simulink model "sm_controlled_current_boost_modificado_renan"  (R2016a)
settings: Solver=VariableStepAuto  StartTime=0.0  StopTime=5  RelTol=1e-3
libraries: powerlib x12
settings Model: Creator=jorda  LastModifiedBy=jorda

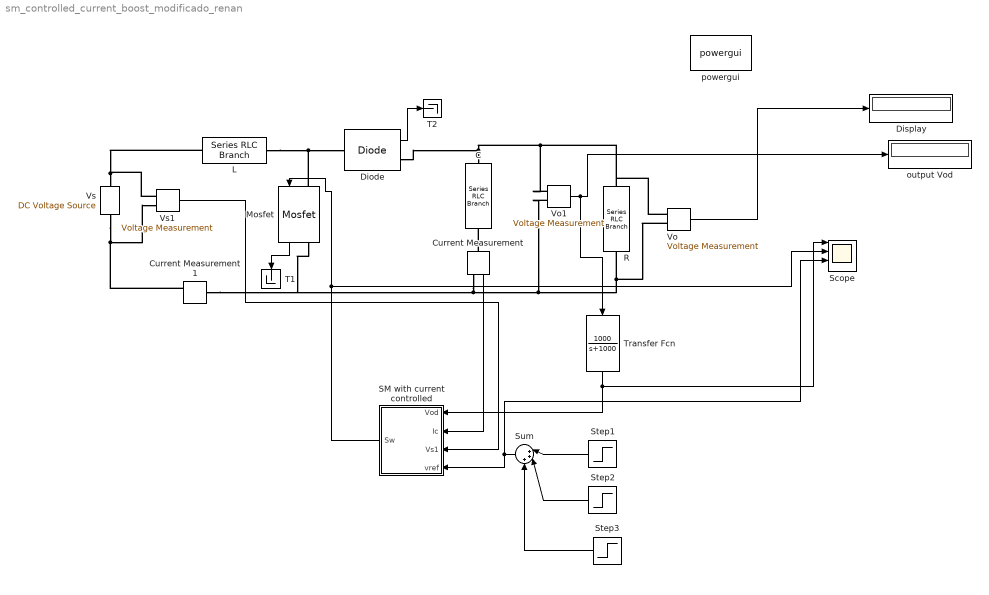
== system sm_controlled_current_boost_modificado_renan ==
  C : powerlib/Elements/Series RLC Branch  LConnTagsString=__new0  RConnTagsString=__new0  BranchType=C  Resistance=1  Inductance=1e-3  SetiL0=off  InitialCurrent=0  Capacitance=2000e-6  Setx0=off  InitialVoltage=0  Measurements=None
  Current Measurement : powerlib/Measurements/Current Measurement  PhasorSimulation=off  OutputType=Complex  PSBequivalent=0
  Current Measurement1 : powerlib/Measurements/Current Measurement  PhasorSimulation=off  OutputType=Complex  PSBequivalent=0
  Diode : powerlib/Power Electronics/Diode  Ron=0.001  Lon=0  Vf=0.8  IC=0  UseSnubber=off  Rs=500  Cs=250e-9  Measurements=on
  Display : Display
  L : powerlib/Elements/Series RLC Branch  LConnTagsString=__new0  RConnTagsString=__new0  BranchType=L  Resistance=1  Inductance=2e-3  SetiL0=off  InitialCurrent=0  Capacitance=1e-6  Setx0=off  InitialVoltage=0  Measurements=None
  Mosfet : powerlib/Power Electronics/Mosfet  Ron=0.1  Lon=0  Rd=0.01  Vfd=0  IC=0  Rs=1e5  Cs=inf  Measurements=on
  R : powerlib/Elements/Series RLC Branch  LConnTagsString=__new0  RConnTagsString=__new0  BranchType=R  Resistance=4  Inductance=1e-3  SetiL0=off  InitialCurrent=0  Capacitance=1e-6  Setx0=off  InitialVoltage=0  Measurements=None
  SM with current controlled : Subsystem
  Scope : Scope  NumInputPorts=4
  Step1 : Step  Before=20  After=22  SampleTime=0
  Step2 : Step  Time=3  After=-2  SampleTime=0
  Step3 : Step  Time=4  Before=3  After=0  SampleTime=0
  Sum : Sum  Inputs=|+++
  T1 : Terminator
  T2 : Terminator
  Transfer Fcn : TransferFcn  Numerator=[1000]  Denominator=[1 1000]
  Vo : powerlib/Measurements/Voltage Measurement  PhasorSimulation=off  OutputType=Complex  PSBequivalent=0
  Vo1 : powerlib/Measurements/Voltage Measurement  PhasorSimulation=off  OutputType=Complex  PSBequivalent=0
  Vs : powerlib/Electrical Sources/DC Voltage Source  Amplitude=15  Measurements=None
  Vs1 : powerlib/Measurements/Voltage Measurement  PhasorSimulation=off  OutputType=Complex  PSBequivalent=0
  output Vod : Display
  powergui : powerlib/powergui  Priority=1  SimulationMode=Continuous  SolverType=Tustin/Backward Euler (TBE)  SampleTime=50e-6  frequency=60  SPID=off  DisableSnubberDevices=off  DisableRonSwitches=off  DisableVfSwitches=off  SwTol=0  DisplayEquations=off  Interpol=off  ExternalGateDelay=off  methode=off  Ts=10  FunctionMessages=off  echomessages=off  HookPort=off  EnableUseOfTLC=off  x0status=blocks  frequencyindice=0  Pbase=100e6  ErrMax=1e-4  Iterations=50  UnitsV=kV  UnitsW=MW  buscounter=0  RestoreLinks=warning  ResistiveCurrentMeasurement=off  Frange=[0:2:500]  Ylog=off  Xlog=on  ShowGrid=off  save=off  variable=ZData  structure=0  ZoomFFT=off  StartTime=0.0  cycles=1  DisplayStyle=1  fundamental=60  FreqAxis=off  MaxFrequency=1000  frequencyindicesteady=1  RmsSteady=1  display=off
  wires:
  Mosfet/1 -> T1/1
  Current Measurement/1 -> SM with current controlled/2(Ic)
  Diode/1 -> T2/1
  SM with current controlled/1(Sw) -> Mosfet/1, Scope/2
  Vs1/1 -> SM with current controlled/3("Vs1 ")
  Step1/1 -> Sum/1
  Sum/1 -> Scope/3, SM with current controlled/4(vref)
  Step2/1 -> Sum/2
  Vo/1 -> Display/1
  Vo1/1 -> Transfer Fcn/1, output Vod/1
  Transfer Fcn/1 -> Scope/1, SM with current controlled/1(Vod)
  Step3/1 -> Sum/3
  connections:
  R/LConn1 -- Vo/LConn1 -- Vo1/LConn1 -- Diode/RConn1 -- C/LConn1
  Current Measurement/RConn1 -- Current Measurement1/LConn1 -- Mosfet/RConn1 -- Vo1/LConn2 -- R/RConn1 -- Vo/LConn2
  Current Measurement/LConn1 -- C/RConn1
  L/RConn1 -- Mosfet/LConn1 -- Diode/LConn1
  Vs/RConn1 -- L/LConn1 -- Vs1/LConn1
  Vs/LConn1 -- Current Measurement1/RConn1 -- Vs1/LConn2

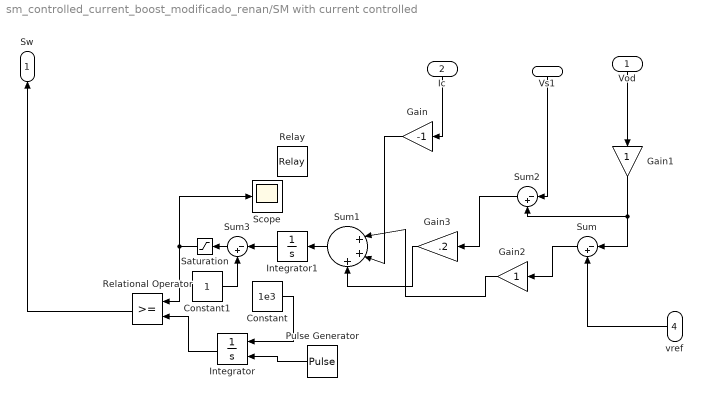
== system sm_controlled_current_boost_modificado_renan/SM with current controlled ==
  Vod : Inport
  Ic : Inport  Port=2
  "Vs1 " : Inport  Port=3
  vref : Inport  Port=4
  Constant : Constant  Value=1e3
  Constant1 : Constant
  Gain : Gain  Gain=-1  ParamDataTypeStr=double  OutDataTypeStr=double
  Gain1 : Gain  ParamDataTypeStr=double  OutDataTypeStr=double
  Gain2 : Gain  ParamDataTypeStr=double  OutDataTypeStr=double
  Gain3 : Gain  Gain=.2  ParamDataTypeStr=double  OutDataTypeStr=double
  Integrator : Integrator  ExternalReset=rising
  Integrator1 : Integrator
  Pulse Generator : DiscretePulseGenerator  PulseType=Time based  Period=1e-3  PulseWidth=.001
  Relational Operator : RelationalOperator  OutDataTypeStr=boolean
  Relay : Relay  OnSwitchValue=0.25  OffSwitchValue=-0.25  OutDataTypeStr=Inherit: Inherit via back propagation
  Saturation : Saturate  UpperLimit=1  LowerLimit=0
  Scope : Scope
  Sum : Sum  Inputs=|-+  AccumDataTypeStr=single  OutDataTypeStr=double  InputSameDT=on
  Sum1 : Sum  Inputs=|+++  AccumDataTypeStr=double  OutDataTypeStr=double  InputSameDT=on
  Sum2 : Sum  Inputs=|-+  AccumDataTypeStr=single  OutDataTypeStr=double  InputSameDT=on
  Sum3 : Sum  Inputs=|-+  AccumDataTypeStr=single  OutDataTypeStr=double  InputSameDT=on
  Sw : Outport
  wires:
  Gain1/1 -> Sum2/2, Sum/1
  Gain/1 -> Sum1/2
  "Vs1 "/1 -> Sum2/1
  Vod/1 -> Gain1/1
  Ic/1 -> Gain/1
  vref/1 -> Sum/2
  Sum2/1 -> Gain3/1
  Sum/1 -> Gain2/1
  Pulse Generator/1 -> Integrator/2
  Constant/1 -> Integrator/1
  Integrator/1 -> Relational Operator/2
  Relational Operator/1 -> Sw/1
  Gain3/1 -> Sum1/3
  Sum1/1 -> Integrator1/1
  Gain2/1 -> Sum1/1
  Integrator1/1 -> Sum3/1
  Constant1/1 -> Sum3/2
  Sum3/1 -> Saturation/1
  Saturation/1 -> Relational Operator/1, Scope/1
